simulink model "simVINS"  (R2018a)
settings: Solver=FixedStepDiscrete  StartTime=0.0  StopTime=inf  FixedStep=1/Fs  RelTol=1e-3  EnableMultiTasking=on
PreLoadFcn:
  | calibrateSFMA=false
  | modelDef = getModelDef(calibrateSFMA);
  | load VINS_bus_definitions.mat;
  | 
  | imuLocationMm = [6 -4.5 -16.8];
  | dejitter_on = true;
  | fidPosUncert = 0.01;
  | 
  | Fs = 1000;  % nominal IMU sampling rate (Hz)
  | 
  | gyroCalBiases = [0;0;0];
  | gyroCalMatrix = eye(3);
  | gyroGsensMatrix = zeros(3,3);
  | Hgyro = [1 0 0 0; 0 1 0 0; 0 0 1 0];
  | 
  | accelCalBiases = [0;0;0];
  | accelCalMatrix = eye(3);
  | Haccel = [1 0 0 0; 0 1 0 0; 0 0 1 0];
  | 
  | imuPar = getImuPar('lmvpCalibrated');
  | optical_cal = getOpticalCalfile();
  | 
  | lastUsedMgyr = zeros(3,3);
  | 
  | 
  | 
  | simData = true;
  | if simData
  |    load truthTrajectory.mat;
  | 
  |    % set Fs based on the timestamps
  |    Fs = 1/mean(diff(truthTrajectory.t.Data));
  |    if Fs>990
  |      Fs = Fs/2;  % bring 1000 Hz down to 500 Hz for faster simulation
  |    end
  | end
  | 
  | imageTensor = uint8(zeros(384,384,2));
  | imageTstamps = 0;
  | useImages = false;
  | useFeatures = false;
  | imageFeatureMatrix = zeros(10,263);
  | 
  | bundle_num_points = 400;
  | bundle_num_frames = 60;
  | 
  | % get rid of following lines if no longer using global data stores to send truth data into VINS
  | truthTraj = Simulink.Signal;
  | truthTraj.DataType = 'Bus: truthTrajectoryBus';
  | truthTraj.InitialValue = '0';
  | truthTraj.Complexity = 'Real';
StartFcn:
  | cd 'C:\Users\efoxlin\Documents\MATLAB\VINS';
undefined symbols (not defined in the file or in its folder): accels, gyros, jumpToXyz, jumpToYaw, tstamp_imu_us, tstamp_vidcap_us, xyz, yaw
libraries: simulink x6, dspmtrx3 x6, dspsrcs4 x6, vrlib x5, dspsigops x2, dspstat3 x2, realtime_pacer_lib x1, dspswit3 x1
(part 1 of 2)
settings Model: Creator=Eric  LastModifiedBy=efoxlin
settings SolverCC: PositivePriorityOrder=on
settings OptimizationCC: DefaultParameterBehavior=Inlined  UseFloatMulNetSlope=on  DefaultUnderspecifiedDataType=single  EnhancedBackFolding=on  PassReuseOutputArgsAs=Individual arguments  EfficientFloat2IntCast=on  MaxStackSize=64  OptimizeBlockOrder=speed  DifferentSizesBufferReuse=on  OptimizationCustomize=off
settings DebuggingCC: SignalInfNanChecking=error  ReadBeforeWriteMsg=DisableAll  WriteAfterWriteMsg=DisableAll  WriteAfterReadMsg=DisableAll  CheckMatrixSingularityMsg=error  ParameterTunabilityLossMsg=error  UnderSpecifiedDataTypeMsg=warning  SignalLabelMismatchMsg=error  UnconnectedOutputMsg=none  BusObjectLabelMismatch=error
settings HardwareCC: ProdBitPerPointer=32  ProdBitPerSizeT=32  ProdBitPerPtrDiffT=32  ProdLargestAtomicInteger=Long  ProdLargestAtomicFloat=Double  ProdWordSize=32  ProdHWDeviceType=ARM Compatible->ARM Cortex
settings SFSimCC: SimParseCustomCode=off  MATLABDynamicMemAlloc=off
settings RTWCC: SystemTargetFile=ert.tlc  GenCodeOnly=on  TemplateMakefile=ert_default_tmf  GenerateReport=on  Toolchain=Microsoft Visual C++ 2017 v15.0 | nmake (64-bit Windows)  BuildConfiguration=Faster Runs  IncludeHyperlinkInReport=on  LaunchReport=on  TargetLang=C++  GenerateTraceInfo=on  GenerateTraceReport=on  GenerateTraceReportSl=on  GenerateTraceReportSf=on  GenerateTraceReportEml=on
settings CodeAppCC: ForceParamTrailComments=on  IgnoreCustomStorageClasses=off  OperatorAnnotations=on  SimulinkDataObjDesc=on  SFDataObjDesc=on  InsertBlockDesc=on
settings ERTTargetCC: TargetLangStandard=C++03 (ISO)  GenerateSampleERTMain=on  MultiInstanceERTCode=on  CodeInterfacePackaging=C++ class  InlinedParameterPlacement=NonHierarchical  RootIOFormat=Structure reference  ERTCustomFileTemplate=example_file_process.tlc

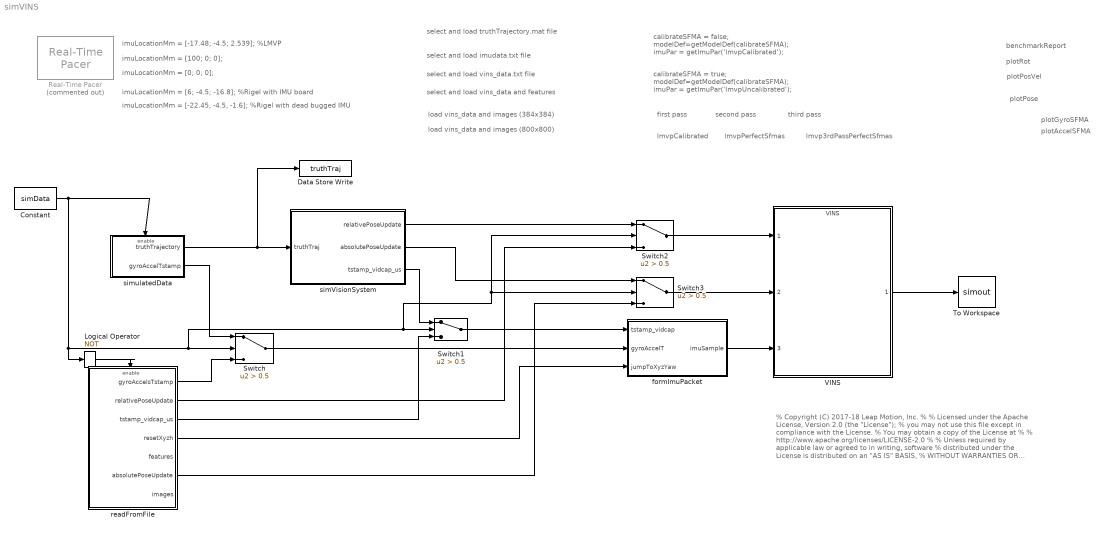
== system simVINS ==
  note: calibrateSFMA = false;
      | modelDef=getModelDef(calibrateSFMA);
      | imuPar = getImuPar('lmvpCalibrated');
  note: imuLocationMm = [-17.48; -4.5; 2.539]; %LMVP
  note: select and load imudata.txt file
  note: second pass
  note: first pass
  note: plotPosVel
  note: plotRot
  note: third pass
  note: select and load truthTrajectory.mat file
  note: lmvpCalibrated
  note: imuLocationMm = [0; 0; 0];
  note: imuLocationMm = [100; 0; 0];
  note: plotPose
  note: lmvpPerfectSfmas
  note: select and load vins_data.txt file
  note: lmvp3rdPassPerfectSfmas
  note: benchmarkReport
  note: calibrateSFMA = true;
      | modelDef=getModelDef(calibrateSFMA);
      | imuPar = getImuPar('lmvpUncalibrated');
  note: plotGyroSFMA
  note: plotAccelSFMA
  note: imuLocationMm = [6; -4.5; -16.8]; %Rigel with IMU board
  note: imuLocationMm = [-22.45, -4.5, -1.6]; %Rigel with dead bugged IMU
  note: select and load vins_data and features
  note: load vins_data and images (800x800)
  note: load vins_data and images (384x384)
  note: % Copyright (C) 2017-18 Leap Motion, Inc.
      | %
      | %    Licensed under the Apache License, Version 2.0 (the "License");
      | %    you may not use this file except in compliance with the License.
      | %    You may obtain a copy of the License at
      | %
      | %        http://www.apache.org/licenses/LICENSE-2.0
      | %
      | %    Unless required by applicable law or agreed to in writing, software
      | %    distributed under the License is distributed on an "AS IS" BASIS,
      | %    WITHOUT WARRANTIES OR CONDITIONS OF ANY KIND, either express or implied.
      | %    See the License for the specific language governing permissions and
      | %    limitations under the License.
      | % Author: Eric Foxlin
  Constant : Constant  Value=simData
  Data Store Write : DataStoreWrite  DataStoreName=truthTraj  DataStoreElements=truthTraj
  Logical Operator : Logic  Operator=NOT  IconShape=distinctive  AllPortsSameDT=off  OutDataTypeStr=boolean
  Real-Time Pacer : realtime_pacer_lib/Real-Time Pacer  Commented=on  simTimePerRealTime=1
  Switch{,1..3} (4 alike) : Switch  Criteria=u2 > Threshold  Threshold=0.5
  To Workspace : ToWorkspace  VariableName=simout  SaveFormat=Timeseries  SampleTime=-1
      settings: Save2DSignal=2-D array (concatenate along first dimension)
  VINS : ModelReference  ModelNameDialog=VINS.slx  SimulationMode=Normal  CodeInterface=Top model  ModelReferenceVersion=1.743
  formImuPacket : Subsystem
  readFromFile : Subsystem
  simVisionSystem : Subsystem  TreatAsAtomicUnit=on
  simulatedData : Subsystem
  wires:
  VINS/1 -> To Workspace/1
  readFromFile/1(gyroAccelsTstamp) -> Switch/3
  simulatedData/2("gyroAccelTstamp ") -> Switch/1
  Constant/1 -> Logical Operator/1, Switch2/2, Switch3/2, Switch1/2, Switch/2, simulatedData/Enable
  Logical Operator/1 -> readFromFile/Enable
  simulatedData/1(truthTrajectory) -> Data Store Write/1, simVisionSystem/1(truthTraj)
  Switch/1 -> formImuPacket/2(gyroAccelT)
  formImuPacket/1(imuSample) -> VINS/3
  simVisionSystem/3(tstamp_vidcap_us) -> Switch1/1
  simVisionSystem/1(relativePoseUpdate) -> Switch2/1
  Switch3/1 -> VINS/2
  Switch1/1 -> formImuPacket/1(tstamp_vidcap)
  readFromFile/3(tstamp_vidcap_us) -> Switch1/3
  Switch2/1 -> VINS/1
  readFromFile/2(relativePoseUpdate) -> Switch2/3
  readFromFile/4(resetXyzh) -> formImuPacket/3(jumpToXyzYaw)
  simVisionSystem/2(absolutePoseUpdate) -> Switch3/1
  readFromFile/6(absolutePoseUpdate) -> Switch3/3

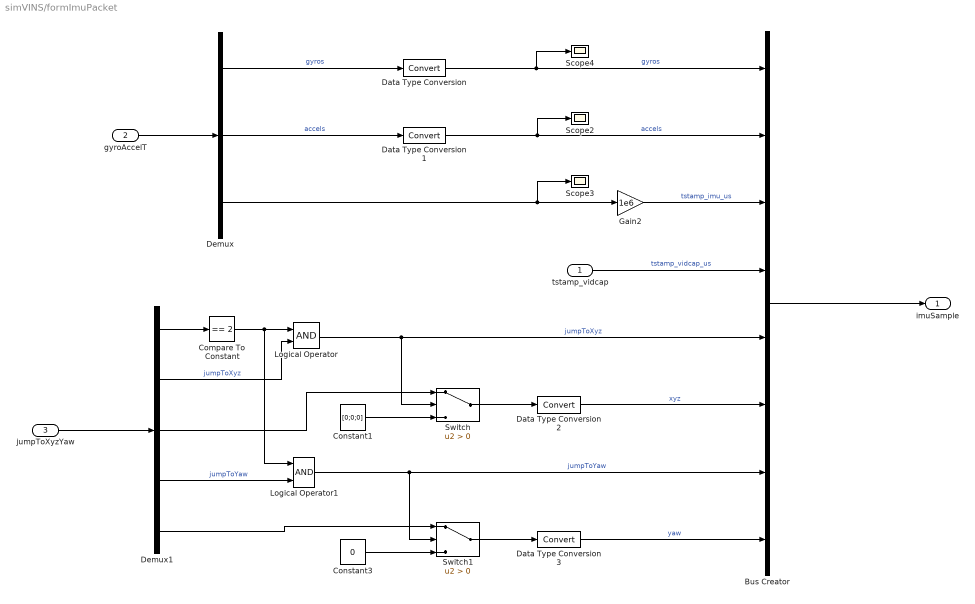
== system simVINS/formImuPacket ==
  tstamp_vidcap : Inport
  gyroAccelT : Inport  Port=2
  jumpToXyzYaw : Inport  Port=3
  Bus Creator : BusCreator  Inputs=gyros,accels,tstamp_imu_us,tstamp_vidcap_us,jumpToXyz,xyz,jumpToYaw,yaw  OutDataTypeStr=Bus: imuSample  NonVirtualBus=on
  Compare To Constant : simulink/Logic and Bit Operations/Compare To Constant  relop===  const=2  OutDataTypeStr=boolean
  Constant1 : Constant  Value=[0;0;0]
  Constant3 : Constant  Value=0
  Data Type Conversion{,1..3} (4 alike) : DataTypeConversion
  Demux : Demux  Outputs=[3 3 1]
  Demux1 : Demux  Outputs=[1 1 3 1 1]
  Gain2 : Gain  Gain=1e6
  Logical Operator : Logic  AllPortsSameDT=off  OutDataTypeStr=boolean
  Logical Operator1 : Logic  AllPortsSameDT=off  OutDataTypeStr=boolean
  Scope2 : Scope
  Scope3 : Scope
  Scope4 : Scope
  Switch : Switch  Criteria=u2 > Threshold
  Switch1 : Switch  Criteria=u2 > Threshold
  imuSample : Outport
  wires:
  Demux/2 -> Data Type Conversion1/1  "accels"
  Demux/1 -> Data Type Conversion/1  "gyros"
  gyroAccelT/1 -> Demux/1
  Bus Creator/1 -> imuSample/1
  Gain2/1 -> Bus Creator/3  "tstamp_imu_us"
  tstamp_vidcap/1 -> Bus Creator/4  "tstamp_vidcap_us"
  Data Type Conversion/1 -> Scope4/1, Bus Creator/1  "gyros"
  Data Type Conversion1/1 -> Scope2/1, Bus Creator/2  "accels"
  Demux/3 -> Gain2/1, Scope3/1
  Logical Operator/1 -> Switch/2, Bus Creator/5  "jumpToXyz"
  Data Type Conversion2/1 -> Bus Creator/6  "xyz"
  Logical Operator1/1 -> Switch1/2, Bus Creator/7  "jumpToYaw"
  Data Type Conversion3/1 -> Bus Creator/8  "yaw"
  jumpToXyzYaw/1 -> Demux1/1
  Demux1/1 -> Compare To Constant/1
  Demux1/2 -> Logical Operator/2  "jumpToXyz"
  Compare To Constant/1 -> Logical Operator1/1, Logical Operator/1
  Demux1/4 -> Logical Operator1/2  "jumpToYaw"
  Demux1/3 -> Switch/1
  Switch/1 -> Data Type Conversion2/1
  Constant1/1 -> Switch/3
  Switch1/1 -> Data Type Conversion3/1
  Demux1/5 -> Switch1/1
  Constant3/1 -> Switch1/3

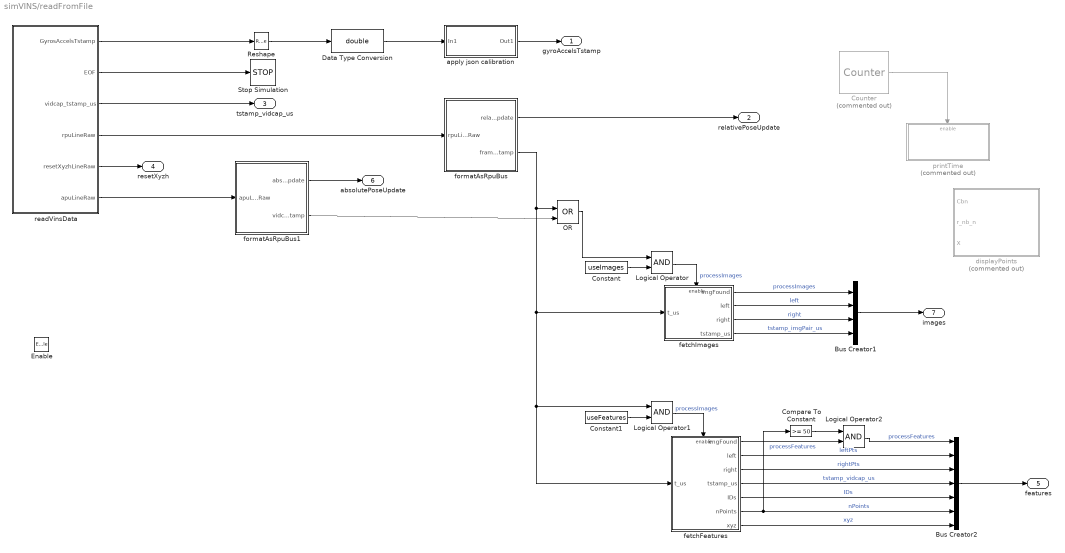
== system simVINS/readFromFile ==
  Enable : EnablePort
  Bus Creator1 : BusCreator  Inputs=4
  Bus Creator2 : BusCreator  Inputs=7
  Compare To Constant : simulink/Logic and Bit Operations/Compare To Constant  relop=>=  const=50  OutDataTypeStr=boolean
  Constant : Constant  Value=useImages
  Constant1 : Constant  Value=useFeatures
  Counter : dspswit3/Counter  Commented=on  Direction=Up  CountEvent=Free running  CounterSize=User defined  MaxCount=4095  InitialCount=0  Output=Hit  HitValue=32  ResetInput=off  SamplesPerFrame=1  Ts=1/Fs  CntDtype=double  HitDtype=Logical
  Data Type Conversion : DataTypeConversion  OutDataTypeStr=double
  Logical Operator : Logic  AllPortsSameDT=off  OutDataTypeStr=boolean
  Logical Operator1 : Logic  AllPortsSameDT=off  OutDataTypeStr=boolean
  Logical Operator2 : Logic  AllPortsSameDT=off  OutDataTypeStr=boolean
  OR : Logic  Operator=OR  IconShape=distinctive  AllPortsSameDT=off  OutDataTypeStr=boolean
  Reshape : Reshape  OutputDimensionality=Column vector (2-D)
  Stop Simulation : Stop
  apply json calibration : Subsystem  TreatAsAtomicUnit=on
  displayPoints : MATLAB Function  Commented=on  TreatAsAtomicUnit=on
  fetchFeatures : Subsystem
  fetchImages : Subsystem
  formatAsRpuBus : Subsystem
  formatAsRpuBus1 : Subsystem
  printTime : Subsystem  Commented=on
  readVinsData : Subsystem
  gyroAccelsTstamp : Outport
  relativePoseUpdate : Outport  Port=2
  tstamp_vidcap_us : Outport  Port=3
  resetXyzh : Outport  Port=4
  features : Outport  Port=5
  absolutePoseUpdate : Outport  Port=6
  images : Outport  Port=7
  wires:
  Reshape/1 -> Data Type Conversion/1
  readVinsData/1(GyrosAccelsTstamp) -> Reshape/1
  readVinsData/2(EOF) -> Stop Simulation/1
  Data Type Conversion/1 -> apply json calibration/1(In1)
  Counter/1 -> printTime/Enable
  apply json calibration/1(Out1) -> gyroAccelsTstamp/1
  readVinsData/3(vidcap_tstamp_us) -> tstamp_vidcap_us/1
  readVinsData/5(resetXyzhLineRaw) -> resetXyzh/1
  fetchImages/2(left) -> Bus Creator1/2  "left"
  fetchImages/3(right) -> Bus Creator1/3  "right"
  Constant/1 -> Logical Operator/2
  Bus Creator1/1 -> images/1
  fetchImages/1(imgFound) -> Bus Creator1/1  "processImages"
  fetchImages/4(tstamp_us) -> Bus Creator1/4  "tstamp_imgPair_us"
  OR/1 -> Logical Operator/1
  readVinsData/4(rpuLineRaw) -> formatAsRpuBus/1(rpuLineRaw)
  formatAsRpuBus/1(relativePoseUpdate) -> relativePoseUpdate/1
  readVinsData/6(apuLineRaw) -> formatAsRpuBus1/1(apuLineRaw)
  formatAsRpuBus1/2(vidcap tstamp) -> OR/2
  Logical Operator/1 -> fetchImages/Enable  "processImages"
  formatAsRpuBus1/1(absolutePoseUpdate) -> absolutePoseUpdate/1
  Logical Operator1/1 -> fetchFeatures/Enable  "processImages"
  formatAsRpuBus/2(frame2 tstamp) -> fetchImages/1(t_us), Logical Operator1/1, fetchFeatures/1(t_us), OR/1
  Constant1/1 -> Logical Operator1/2
  Logical Operator2/1 -> Bus Creator2/1  "processFeatures"
  fetchFeatures/2(left) -> Bus Creator2/2  "leftPts"
  fetchFeatures/3(right) -> Bus Creator2/3  "rightPts"
  fetchFeatures/4(tstamp_us) -> Bus Creator2/4  "tstamp_vidcap_us"
  Bus Creator2/1 -> features/1
  fetchFeatures/5(IDs) -> Bus Creator2/5  "IDs"
  fetchFeatures/6(nPoints) -> Compare To Constant/1, Bus Creator2/6  "nPoints"
  fetchFeatures/7(xyz) -> Bus Creator2/7  "xyz"
  fetchFeatures/1(imgFound) -> Logical Operator2/2  "processFeatures"
  Compare To Constant/1 -> Logical Operator2/1

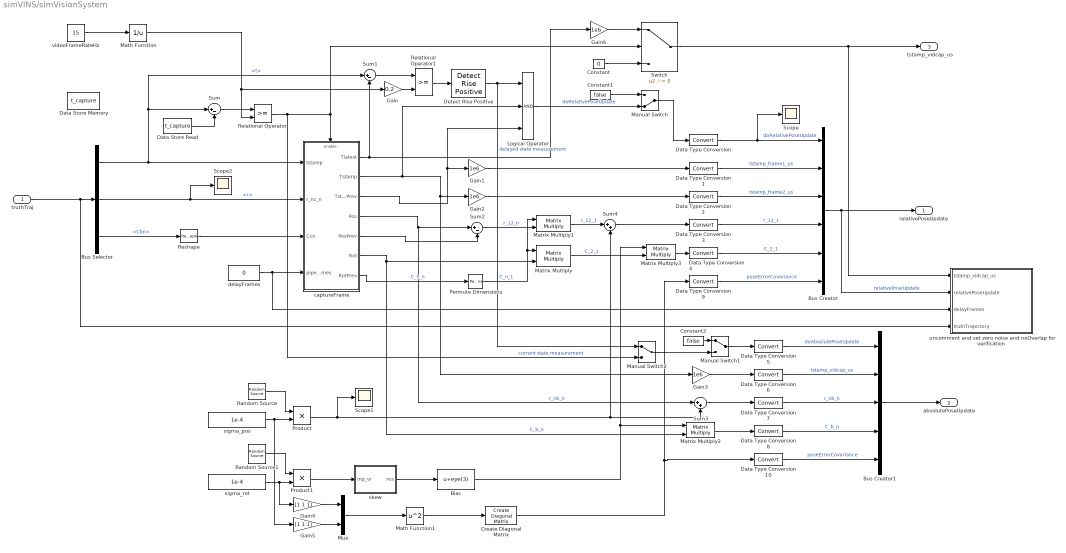
== system simVINS/simVisionSystem ==
  truthTraj : Inport
  Bias : Bias  Bias=eye(3)
  Bus Creator : BusCreator  Inputs=6  OutDataTypeStr=Bus: relativePoseUpdate  NonVirtualBus=on
  Bus Creator1 : BusCreator  Inputs=5  OutDataTypeStr=Bus: absolutePoseUpdate  NonVirtualBus=on
  Bus Selector : BusSelector  OutputSignals=t,r,Cbn
  Constant : Constant  Value=0
  Constant1 : Constant  Value=false
  Constant2 : Constant  Value=false
  Create Diagonal Matrix : dspmtrx3/Create Diagonal Matrix
      settings: SourceProductName=DSP System Toolbox  SourceProductBaseCode=DS
  Data Store Memory : DataStoreMemory  DataStoreName=t_capture  ReadBeforeWriteMsg=warning  WriteAfterWriteMsg=warning  WriteAfterReadMsg=warning  ShowAdditionalParam=off
  Data Store Read : DataStoreRead  DataStoreName=t_capture
  Data Type Conversion{,1..10} (11 alike) : DataTypeConversion
  Detect Rise Positive : simulink/Logic and Bit Operations/Detect Rise Positive  vinit=0  OutDataTypeStr=boolean
  Gain : Gain  Gain=0.2
  Gain{1..3,6} (4 alike) : Gain  Gain=1e6
  Gain4 : Gain  Gain=[1 1 1]
  Gain5 : Gain  Gain=[1 1 1]
  Logical Operator : Logic  Inputs=3  AllPortsSameDT=off  OutDataTypeStr=boolean
  Manual Switch : ManualSwitch  CurrentSetting=0
  Manual Switch1 : ManualSwitch
  Manual Switch2 : ManualSwitch
  Math Function : Math  Operator=reciprocal  SaturateOnIntegerOverflow=on
  Math Function1 : Math  Operator=square  SaturateOnIntegerOverflow=on
  Matrix Multiply{,1..3} (4 alike) : Product  Multiplication=Matrix(*)
  Mux : Mux  Inputs=2
  Permute Dimensions : PermuteDimensions
  Product : Product
  Product1 : Product
  Random Source : dspsrcs4/Random Source  SrcType=Gaussian  NormMethod=Ziggurat  CltLength=12  MinVal=0  MaxVal=1  MeanVal=[0; 0 ; 0]  VarVal=1  RepMode=Not repeatable  rawSeed=1  IsInherit=off  SampMode=Discrete  SampTime=1/Fs  SampFrame=1  DataType=Double  OutComplex=Real  OutputFrames=off
  Random Source1 : dspsrcs4/Random Source  SrcType=Gaussian  NormMethod=Ziggurat  CltLength=12  MinVal=0  MaxVal=1  MeanVal=[0; 0 ; 0]  VarVal=1  RepMode=Not repeatable  rawSeed=1  IsInherit=off  SampMode=Discrete  SampTime=1/Fs  SampFrame=1  DataType=Double  OutComplex=Real  OutputFrames=off
  Relational Operator : RelationalOperator  OutDataTypeStr=boolean  RndMeth=Simplest
  Relational Operator1 : RelationalOperator  OutDataTypeStr=boolean  RndMeth=Simplest
  Reshape : Reshape  OutputDimensionality=Customize  OutputDimensions=[3,3]
  Scope : Scope
  Scope1 : Scope
  Scope2 : Scope
  Sum : Sum  Inputs=|+-
  Sum1 : Sum  Inputs=|+-
  Sum2 : Sum  Inputs=|+-
  Sum3 : Sum  Inputs=|++
  Sum4 : Sum  Inputs=|++
  Switch : Switch  Criteria=u2 ~= 0
  captureFrame : Subsystem  TreatAsAtomicUnit=on
  delayFrames : Constant  Value=0
  sigma_pos : Constant  Value=1e-4
  sigma_rot : Constant  Value=1e-4
  skew : MATLAB Function  TreatAsAtomicUnit=on
  uncomment and set zero noise and noOverlap for verification : Subsystem  TreatAsAtomicUnit=on
  videoFrameRateHz : Constant  Value=15
  relativePoseUpdate : Outport
  absolutePoseUpdate : Outport  Port=2
  tstamp_vidcap_us : Outport  Port=3
  wires:
  truthTraj/1 -> uncomment and set zero noise and noOverlap for verification/4(truthTrajectory), Bus Selector/1
  Bus Selector/1 -> Sum/1, Sum1/1, captureFrame/1(tstamp)  "<t>"
  Sum/1 -> Relational Operator/1
  videoFrameRateHz/1 -> Math Function/1
  Math Function/1 -> Relational Operator/2, Gain/1
  Relational Operator/1 -> Manual Switch2/2, Switch/2, captureFrame/Enable  "current state measurement"
  Bus Selector/2 -> Scope2/1, captureFrame/2(r_nc_n)  "<r>"
  Bus Selector/3 -> Reshape/1  "<Cbn>"
  captureFrame/4(Pos) -> Sum3/1, Sum2/1  "r_nb_n"
  captureFrame/6(Rot) -> Matrix Multiply2/2, Matrix Multiply/2  "C_b_n"
  Sum1/1 -> Relational Operator1/1
  Gain/1 -> Relational Operator1/2
  Relational Operator1/1 -> Detect Rise Positive/1
  captureFrame/3(TstampPrev) -> Logical Operator/3, Gain1/1
  Manual Switch/1 -> Data Type Conversion/1
  captureFrame/2(Tstamp) -> Logical Operator/2, Gain3/1, Gain2/1
  captureFrame/5(PosPrev) -> Sum2/2
  Sum2/1 -> Matrix Multiply1/2  "r_12_n"
  Reshape/1 -> captureFrame/3(Ccn)
  Matrix Multiply3/1 -> Data Type Conversion4/1
  captureFrame/7(RotPrev) -> Permute Dimensions/1  "C_1_n"
  Permute Dimensions/1 -> Matrix Multiply1/1, Matrix Multiply/1  "C_n_1"
  Bus Creator/1 -> relativePoseUpdate/1, uncomment and set zero noise and noOverlap for verification/2(relativePoseUpdate)  "relativePoseUpdate"
  Sum4/1 -> Data Type Conversion3/1
  Gain1/1 -> Data Type Conversion1/1
  Gain2/1 -> Data Type Conversion2/1
  Data Store Read/1 -> Sum/2
  Switch/1 -> tstamp_vidcap_us/1, uncomment and set zero noise and noOverlap for verification/1(tstamp_vidcap_us)
  Constant/1 -> Switch/3
  Detect Rise Positive/1 -> Logical Operator/1, Manual Switch2/1  "delayed state measurement"
  Logical Operator/1 -> Manual Switch/2  "doRelativePoseUpdate"
  Constant1/1 -> Manual Switch/1
  Bus Creator1/1 -> absolutePoseUpdate/1
  Constant2/1 -> Manual Switch1/1
  Manual Switch1/1 -> Data Type Conversion5/1
  Gain3/1 -> Data Type Conversion6/1
  Sum3/1 -> Data Type Conversion7/1
  Matrix Multiply2/1 -> Data Type Conversion8/1
  sigma_pos/1 -> Gain5/1, Product/2
  Random Source/1 -> Product/1
  Random Source1/1 -> Product1/1
  sigma_rot/1 -> Gain4/1, Product1/2
  Product1/1 -> skew/1(inp_vr)
  skew/1(res) -> Bias/1
  Manual Switch2/1 -> Manual Switch1/2
  Bias/1 -> Matrix Multiply3/1, Matrix Multiply2/1
  Matrix Multiply1/1 -> Sum4/1  "r_12_1"
  Matrix Multiply/1 -> Matrix Multiply3/2  "C_2_1"
  Data Type Conversion/1 -> Scope/1, Bus Creator/1  "doRelativePoseUpdate"
  Data Type Conversion1/1 -> Bus Creator/2  "tstamp_frame1_us"
  Data Type Conversion2/1 -> Bus Creator/3  "tstamp_frame2_us"
  Data Type Conversion3/1 -> Bus Creator/4  "r_12_1"
  Data Type Conversion4/1 -> Bus Creator/5  "C_2_1"
  Data Type Conversion5/1 -> Bus Creator1/1  "doAbsolutePoseUpdate"
  Data Type Conversion6/1 -> Bus Creator1/2  "tstamp_vidcap_us"
  Data Type Conversion7/1 -> Bus Creator1/3  "r_nb_n"
  Data Type Conversion8/1 -> Bus Creator1/4  "C_b_n"
  Gain4/1 -> Mux/1
  Gain5/1 -> Mux/2
  Mux/1 -> Math Function1/1
  Data Type Conversion9/1 -> Bus Creator/6  "poseErrorCovariance"
  Data Type Conversion10/1 -> Bus Creator1/5  "poseErrorCovariance"
  Create Diagonal Matrix/1 -> Data Type Conversion10/1, Data Type Conversion9/1
  Math Function1/1 -> Create Diagonal Matrix/1
  delayFrames/1 -> uncomment and set zero noise and noOverlap for verification/3(delayFrames), captureFrame/4(pipelineDelayFrames)
  captureFrame/1(Tlatest) -> Gain6/1, Sum1/2
  Gain6/1 -> Switch/1
  Product/1 -> Scope1/1, Sum4/2, Sum3/2

== system simVINS/simulatedData ==
  note: truthTrajectory is motion of the camera device frame with origin
      | halfway between two lenses.
      | VINS tracking is done in body frame of IMU, which is offset
      | by imuLocationMm,  but output is converted to device frame.
  Enable : EnablePort
  From Workspace : FromWorkspace  VariableName=truthTrajectory  OutDataTypeStr=Bus: truthTrajectoryBus  SampleTime=1/Fs  Interpolate=off  OutputAfterFinalValue=Setting to zero
  To Workspace1 : ToWorkspace  VariableName=truthout  SaveFormat=Timeseries  SampleTime=-1
      settings: Save2DSignal=2-D array (concatenate along first dimension)
  reportOutputs : Subsystem  Priority=10  TreatAsAtomicUnit=on
  simulateIdealImuWithOffset : Subsystem
  simulateImuErrors : Subsystem  TreatAsAtomicUnit=on
  "t, rpy, PQR, rnav, vnav, anav way too slow!" : FromFile  Commented=on  FileName=truthTrajectory.mat  OutDataTypeStr=Bus: truthTrajectoryBus  SampleTime=1/Fs  ExtrapolationBeforeFirstDataPoint=Ground value  InterpolationWithinTimeRange=Zero order hold  ExtrapolationAfterLastDataPoint=Ground value
  uncomment for INS integration verification : Subsystem  TreatAsAtomicUnit=on
  truthTrajectory : Outport
  "gyroAccelTstamp " : Outport  Port=2
  wires:
  simulateIdealImuWithOffset/1(gyrosAccelsTstamp) -> uncomment for INS integration verification/1(gyroAccelT), simulateImuErrors/1(gyroAccelT)
  From Workspace/1 -> truthTrajectory/1, reportOutputs/1(truthTraj), uncomment for INS integration verification/2(truthTrajectory), simulateIdealImuWithOffset/1(In1)
  reportOutputs/1(truthOut) -> To Workspace1/1
  simulateImuErrors/5(withErrors) -> "gyroAccelTstamp "/1
  simulateImuErrors/1(gyroBias) -> reportOutputs/2(truth dw)
  simulateImuErrors/2(accelBias) -> reportOutputs/3(truth df)

== system simVINS/readFromFile/apply json calibration ==
  note: if there is a .json file in the directory where imudata.txt file had been stored,
      | it gets parsed during file load to produce the homogeneous 3x4 matrices Hgyro and Haccel.
      | If not, these are set to identity with no biases so that they don't do anything.
  In1 : Inport
  Constant : Constant  Value=Hgyro
  Constant1 : Constant  Value=Haccel
  Demux : Demux  Outputs=[3 3 1]
  Mux : Mux  Inputs=3
  Product : Product  Multiplication=Matrix(*)
  Product1 : Product  Multiplication=Matrix(*)
  Reshape : Reshape  OutputDimensionality=Column vector (2-D)
  Reshape1 : Reshape  OutputDimensionality=Column vector (2-D)
  add a 1 as fourth element for homogeneous multiply : dspsigops/Pad  padAlong=Columns  dimsToPad=1  valSrc=Specify via dialog  padVal=1  spec=Output size  padNumOutRowsSpecMethod=User-specified  numOutRows=4  padNumOutColsSpecMethod=User-specified  numOutCols=1  isVarDimsMode=off  padBeginning=0  padEnd=0  outSizeMode=User-specified  outSize=1  padSigAt=End  trunc_flag=None  roundingMode=Floor  overflowMode=off  truncOrWrapMode=Truncate  wrap_flag=None
      settings: SourceProductName=DSP System Toolbox  SourceProductBaseCode=DS
  add a 1 as fourth element for homogeneous multiply1 : dspsigops/Pad  padAlong=Columns  dimsToPad=1  valSrc=Specify via dialog  padVal=1  spec=Output size  padNumOutRowsSpecMethod=User-specified  numOutRows=4  padNumOutColsSpecMethod=User-specified  numOutCols=1  isVarDimsMode=off  padBeginning=0  padEnd=0  outSizeMode=User-specified  outSize=1  padSigAt=End  trunc_flag=None  roundingMode=Floor  overflowMode=off  truncOrWrapMode=Truncate  wrap_flag=None
      settings: SourceProductName=DSP System Toolbox  SourceProductBaseCode=DS
  Out1 : Outport
  wires:
  In1/1 -> Demux/1
  Demux/1 -> Reshape/1
  Constant/1 -> Product/1
  Demux/2 -> Reshape1/1
  Constant1/1 -> Product1/1
  Product/1 -> Mux/1
  Product1/1 -> Mux/2
  Mux/1 -> Out1/1
  Reshape/1 -> add a 1 as fourth element for homogeneous multiply/1
  Reshape1/1 -> add a 1 as fourth element for homogeneous multiply1/1
  add a 1 as fourth element for homogeneous multiply/1 -> Product/2
  add a 1 as fourth element for homogeneous multiply1/1 -> Product1/2
  Demux/3 -> Mux/3

== system simVINS/readFromFile/fetchFeatures ==
  t_us : Inport
  Enable : EnablePort  PropagateVarSize=During execution
  Constant : Constant  Value=imageFeatureMatrix
  Display1 : Display
  MATLAB Function : MATLAB Function  TreatAsAtomicUnit=on
  Scope : Scope
  getImgNum : Subsystem  Priority=1
  imgFound : Outport  OutputWhenDisabled=reset  InitialOutput=false
  left : Outport  Port=2
  right : Outport  Port=3
  tstamp_us : Outport  Port=4  OutputWhenDisabled=reset  InitialOutput=0
  IDs : Outport  Port=5
  nPoints : Outport  Port=6
  xyz : Outport  Port=7
  wires:
  getImgNum/2(imgFound) -> imgFound/1
  t_us/1 -> getImgNum/1(t_us), tstamp_us/1
  MATLAB Function/4(rightPts) -> right/1
  Constant/1 -> MATLAB Function/2(imageFeatureMatrix)
  getImgNum/1(imgNum) -> Scope/1, MATLAB Function/1(imgNum)
  MATLAB Function/3(leftPts) -> left/1
  MATLAB Function/2(IDs) -> IDs/1
  MATLAB Function/1(nPoints) -> Display1/1, nPoints/1
  MATLAB Function/5(xyz) -> xyz/1

== system simVINS/readFromFile/fetchImages ==
  t_us : Inport
  Enable : EnablePort
  Constant : Constant  Value=imageTensor
  MATLAB Function : MATLAB Function  TreatAsAtomicUnit=on
  Scope : Scope
  getImgNum : Subsystem  Priority=1
  imgFound : Outport  OutputWhenDisabled=reset  InitialOutput=false
  left : Outport  Port=2
  right : Outport  Port=3
  tstamp_us : Outport  Port=4  OutputWhenDisabled=reset  InitialOutput=0
  wires:
  MATLAB Function/1(left) -> left/1
  getImgNum/1(imgNum) -> MATLAB Function/1(imgNum), Scope/1
  Constant/1 -> MATLAB Function/2(imageTensor)
  MATLAB Function/2(right) -> right/1
  t_us/1 -> tstamp_us/1, getImgNum/1(t_us)
  getImgNum/2(imgFound) -> imgFound/1

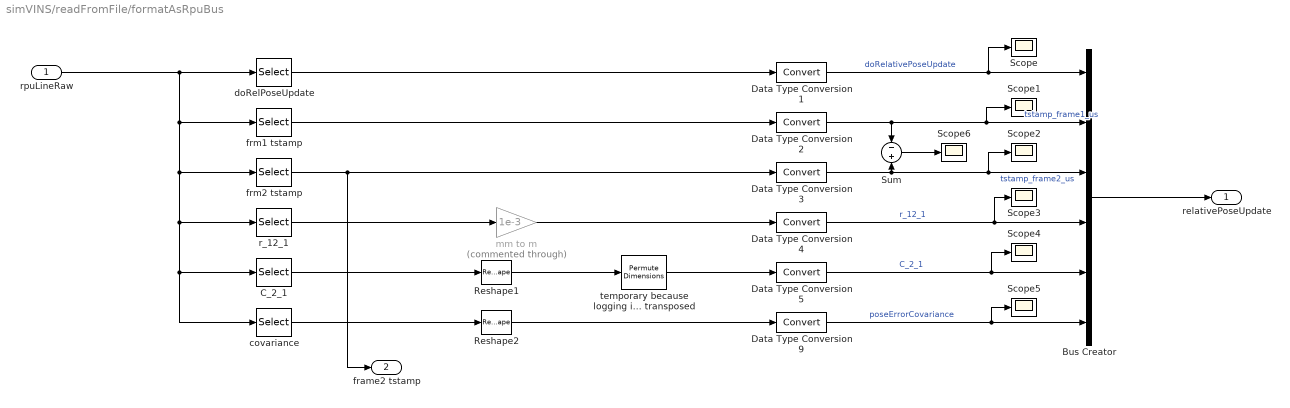
== system simVINS/readFromFile/formatAsRpuBus ==
  rpuLineRaw : Inport
  Bus Creator : BusCreator  Inputs=6  OutDataTypeStr=Bus: relativePoseUpdate  NonVirtualBus=on
  C_2_1 : Selector  InputPortWidth=52  IndexOptions=Index vector (dialog)  Indices=4:12  OutputSizes=1
  Data Type Conversion{1..5,9} (6 alike) : DataTypeConversion
  Reshape1 : Reshape  OutputDimensionality=Customize  OutputDimensions=[3,3]
  Reshape2 : Reshape  OutputDimensionality=Customize  OutputDimensions=[6,6]
  Scope{,1..6} (7 alike) : Scope
  Sum : Sum  Inputs=-+
  covariance : Selector  InputPortWidth=52  IndexOptions=Index vector (dialog)  Indices=16:51  OutputSizes=1
  doRelPoseUpdate : Selector  InputPortWidth=52  IndexOptions=Index vector (dialog)  Indices=52  OutputSizes=1
  frm1 tstamp : Selector  InputPortWidth=52  IndexOptions=Index vector (dialog)  Indices=2  OutputSizes=1
  frm2 tstamp : Selector  InputPortWidth=52  IndexOptions=Index vector (dialog)  Indices=3  OutputSizes=1
  mm to m : Gain  Commented=through  Gain=1e-3
  r_12_1 : Selector  InputPortWidth=52  IndexOptions=Index vector (dialog)  Indices=13:15  OutputSizes=1
  temporary because logging is transposed : PermuteDimensions
  relativePoseUpdate : Outport
  frame2 tstamp : Outport  Port=2
  wires:
  Sum/1 -> Scope6/1
  Data Type Conversion3/1 -> Sum/2, Bus Creator/3, Scope2/1  "tstamp_frame2_us"
  rpuLineRaw/1 -> frm1 tstamp/1, frm2 tstamp/1, r_12_1/1, C_2_1/1, covariance/1, doRelPoseUpdate/1
  Reshape1/1 -> temporary because logging is transposed/1
  C_2_1/1 -> Reshape1/1
  Data Type Conversion9/1 -> Scope5/1, Bus Creator/6  "poseErrorCovariance"
  doRelPoseUpdate/1 -> Data Type Conversion1/1
  Data Type Conversion2/1 -> Sum/1, Scope1/1, Bus Creator/2  "tstamp_frame1_us"
  Data Type Conversion5/1 -> Scope4/1, Bus Creator/5  "C_2_1"
  r_12_1/1 -> mm to m/1
  frm2 tstamp/1 -> frame2 tstamp/1, Data Type Conversion3/1
  Data Type Conversion1/1 -> Scope/1, Bus Creator/1  "doRelativePoseUpdate"
  temporary because logging is transposed/1 -> Data Type Conversion5/1
  Reshape2/1 -> Data Type Conversion9/1
  Data Type Conversion4/1 -> Scope3/1, Bus Creator/4  "r_12_1"
  frm1 tstamp/1 -> Data Type Conversion2/1
  covariance/1 -> Reshape2/1
  mm to m/1 -> Data Type Conversion4/1
  Bus Creator/1 -> relativePoseUpdate/1

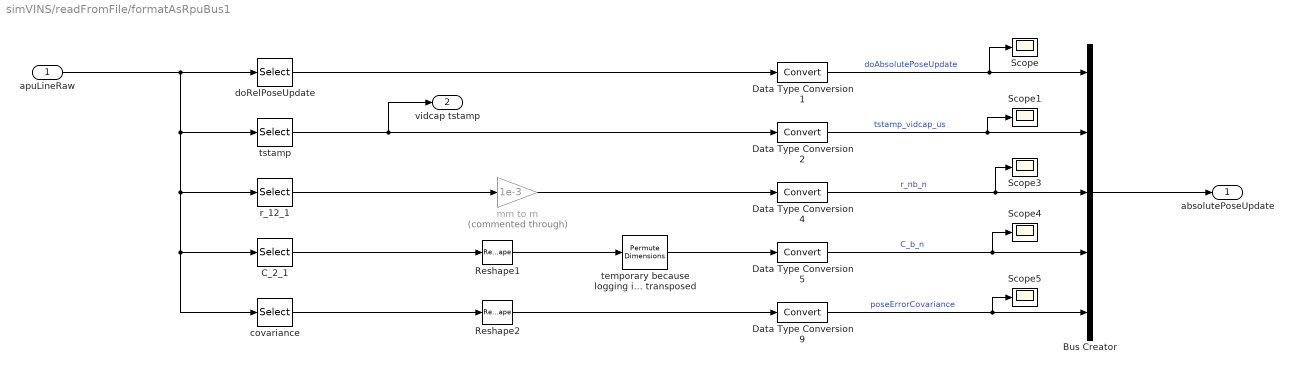
== system simVINS/readFromFile/formatAsRpuBus1 ==
  apuLineRaw : Inport
  " tstamp" : Selector  InputPortWidth=51  IndexOptions=Index vector (dialog)  Indices=2  OutputSizes=1
  Bus Creator : BusCreator  Inputs=5  OutDataTypeStr=Bus: absolutePoseUpdate  NonVirtualBus=on
  C_2_1 : Selector  InputPortWidth=51  IndexOptions=Index vector (dialog)  Indices=3:11  OutputSizes=1
  Data Type Conversion{1..2,4..5,9} (5 alike) : DataTypeConversion
  Reshape1 : Reshape  OutputDimensionality=Customize  OutputDimensions=[3,3]
  Reshape2 : Reshape  OutputDimensionality=Customize  OutputDimensions=[6,6]
  Scope{,1,3..5} (5 alike) : Scope
  covariance : Selector  InputPortWidth=51  IndexOptions=Index vector (dialog)  Indices=15:50  OutputSizes=1
  doRelPoseUpdate : Selector  InputPortWidth=51  IndexOptions=Index vector (dialog)  Indices=51  OutputSizes=1
  mm to m : Gain  Commented=through  Gain=1e-3
  r_12_1 : Selector  InputPortWidth=51  IndexOptions=Index vector (dialog)  Indices=12:14  OutputSizes=1
  temporary because logging is transposed : PermuteDimensions
  absolutePoseUpdate : Outport
  vidcap tstamp : Outport  Port=2
  wires:
  Bus Creator/1 -> absolutePoseUpdate/1
  mm to m/1 -> Data Type Conversion4/1
  covariance/1 -> Reshape2/1
  " tstamp"/1 -> vidcap tstamp/1, Data Type Conversion2/1
  Data Type Conversion4/1 -> Bus Creator/3, Scope3/1  "r_nb_n"
  Reshape2/1 -> Data Type Conversion9/1
  temporary because logging is transposed/1 -> Data Type Conversion5/1
  Data Type Conversion1/1 -> Bus Creator/1, Scope/1  "doAbsolutePoseUpdate"
  r_12_1/1 -> mm to m/1
  Data Type Conversion5/1 -> Bus Creator/4, Scope4/1  "C_b_n"
  Data Type Conversion2/1 -> Bus Creator/2, Scope1/1  "tstamp_vidcap_us"
  doRelPoseUpdate/1 -> Data Type Conversion1/1
  Data Type Conversion9/1 -> Bus Creator/5, Scope5/1  "poseErrorCovariance"
  C_2_1/1 -> Reshape1/1
  Reshape1/1 -> temporary because logging is transposed/1
  apuLineRaw/1 -> covariance/1, C_2_1/1, r_12_1/1, " tstamp"/1, doRelPoseUpdate/1

== system simVINS/readFromFile/printTime ==
  Enable : EnablePort
  Digital Clock : DigitalClock  SampleTime=1/Fs
  MATLAB Function : MATLAB Function  TreatAsAtomicUnit=on
  wires:
  Digital Clock/1 -> MATLAB Function/1(u)

== system simVINS/readFromFile/readVinsData ==
  C++ S-function : S-Function  FunctionName=readVinsData  Parameters=1/Fs  SFunctionDeploymentMode=off  EnableBusSupport=off
  Gain : Gain  Gain=1e-6
  Mux : Mux  Inputs=[3 3 1]
  Unit Delay : UnitDelay  SampleTime=-1
  accels : Selector  InputPortWidth=10  IndexOptions=Index vector (dialog)  Indices=3:5  OutputSizes=1
  avoid sending garbage on the last row : Switch  Criteria=u2 > Threshold  Threshold=0.5
  gyros : Selector  InputPortWidth=10  IndexOptions=Index vector (dialog)  Indices=6:8  OutputSizes=1
  t_us : Selector  InputPortWidth=10  IndexOptions=Index vector (dialog)  Indices=2  OutputSizes=1
  vidcap_tstamp : Selector  InputPortWidth=10  IndexOptions=Index vector (dialog)  Indices=9  OutputSizes=1
  GyrosAccelsTstamp : Outport
  EOF : Outport  Port=2
  vidcap_tstamp_us : Outport  Port=3
  rpuLineRaw : Outport  Port=4
  resetXyzhLineRaw : Outport  Port=5
  apuLineRaw : Outport  Port=6
  wires:
  C++ S-function/1 -> t_us/1, gyros/1, accels/1, vidcap_tstamp/1
  Mux/1 -> Unit Delay/1, avoid sending garbage on the last row/3
  avoid sending garbage on the last row/1 -> GyrosAccelsTstamp/1
  Unit Delay/1 -> avoid sending garbage on the last row/1
  C++ S-function/5 -> avoid sending garbage on the last row/2, EOF/1
  C++ S-function/2 -> rpuLineRaw/1
  vidcap_tstamp/1 -> vidcap_tstamp_us/1
  gyros/1 -> Mux/1
  accels/1 -> Mux/2
  t_us/1 -> Gain/1
  Gain/1 -> Mux/3
  C++ S-function/3 -> resetXyzhLineRaw/1
  C++ S-function/4 -> apuLineRaw/1

== system simVINS/simVisionSystem/captureFrame ==
  tstamp : Inport
  r_nc_n : Inport  Port=2
  Ccn : Inport  Port=3
  pipelineDelayFrames : Inport  Port=4
  Enable : EnablePort
  Data Store Write : DataStoreWrite  DataStoreName=t_capture
  Delay : Delay  DelayLengthSource=Input port
      settings: InputPortMap=u0,p1
  Delay1 : Delay  DelayLengthSource=Input port
      settings: InputPortMap=u0,p1
  Delay2 : Delay  DelayLengthSource=Input port
      settings: InputPortMap=u0,p1
  Unit Delay3 : UnitDelay  SampleTime=-1
  Unit Delay4 : UnitDelay  SampleTime=-1
  Unit Delay5 : UnitDelay  SampleTime=-1
  Tlatest : Outport
  Tstamp : Outport  Port=2
  TstampPrev : Outport  Port=3
  Pos : Outport  Port=4
  PosPrev : Outport  Port=5
  Rot : Outport  Port=6
  RotPrev : Outport  Port=7
  wires:
  tstamp/1 -> Data Store Write/1, Delay/1, Tlatest/1
  Ccn/1 -> Delay2/1  "Cbn"
  Delay/1 -> Unit Delay3/1, Tstamp/1
  Unit Delay3/1 -> TstampPrev/1
  r_nc_n/1 -> Delay1/1
  Delay1/1 -> Unit Delay4/1, Pos/1
  Unit Delay4/1 -> PosPrev/1
  Delay2/1 -> Unit Delay5/1, Rot/1
  Unit Delay5/1 -> RotPrev/1
  pipelineDelayFrames/1 -> Delay2/2, Delay1/2, Delay/2

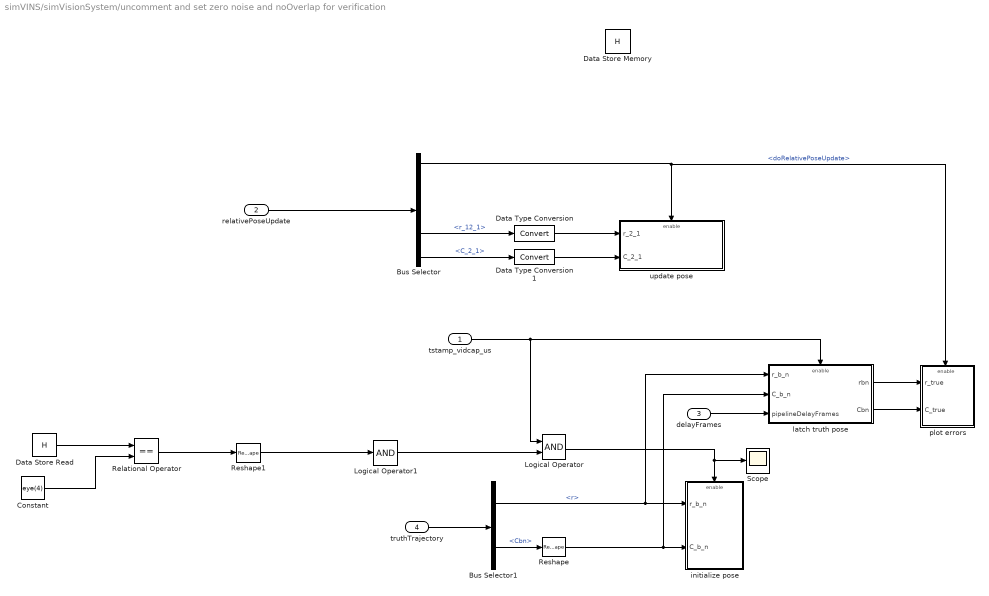
== system simVINS/simVisionSystem/uncomment and set zero noise and noOverlap for verification ==
  tstamp_vidcap_us : Inport
  relativePoseUpdate : Inport  Port=2
  delayFrames : Inport  Port=3
  truthTrajectory : Inport  Port=4
  Bus Selector : BusSelector  OutputSignals=doRelativePoseUpdate,tstamp_frame1_us,tstamp_frame2_us,r_12_1,C_2_1
  Bus Selector1 : BusSelector  OutputSignals=r,Cbn
  Constant : Constant  Value=eye(4)
  Data Store Memory : DataStoreMemory  DataStoreName=H  ReadBeforeWriteMsg=warning  WriteAfterWriteMsg=warning  WriteAfterReadMsg=warning  InitialValue=eye(4)  ShowAdditionalParam=off
  Data Store Read : DataStoreRead  DataStoreName=H
  Data Type Conversion : DataTypeConversion
  Data Type Conversion1 : DataTypeConversion
  Logical Operator : Logic  AllPortsSameDT=off  OutDataTypeStr=boolean
  Logical Operator1 : Logic  Inputs=1  AllPortsSameDT=off  OutDataTypeStr=boolean
  Relational Operator : RelationalOperator  Operator===  OutDataTypeStr=boolean  RndMeth=Simplest
  Reshape : Reshape  OutputDimensionality=Customize  OutputDimensions=[3,3]
  Reshape1 : Reshape
  Scope : Scope
  initialize pose : Subsystem  TreatAsAtomicUnit=on
  latch truth pose : Subsystem  TreatAsAtomicUnit=on
  plot errors : Subsystem  TreatAsAtomicUnit=on
  update pose : Subsystem  TreatAsAtomicUnit=on
  wires:
  relativePoseUpdate/1 -> Bus Selector/1
  Bus Selector/1 -> plot errors/Enable, update pose/Enable  "<doRelativePoseUpdate>"
  Bus Selector/4 -> Data Type Conversion/1  "<r_12_1>"
  Bus Selector/5 -> Data Type Conversion1/1  "<C_2_1>"
  truthTrajectory/1 -> Bus Selector1/1
  Bus Selector1/1 -> latch truth pose/1(r_b_n), initialize pose/1(r_b_n)  "<r>"
  Bus Selector1/2 -> Reshape/1  "<Cbn>"
  Logical Operator/1 -> Scope/1, initialize pose/Enable
  Data Store Read/1 -> Relational Operator/1
  Constant/1 -> Relational Operator/2
  Relational Operator/1 -> Reshape1/1
  tstamp_vidcap_us/1 -> latch truth pose/Enable, Logical Operator/1
  Reshape/1 -> latch truth pose/2(C_b_n), initialize pose/2(C_b_n)
  latch truth pose/1(rbn) -> plot errors/1(r_true)
  latch truth pose/2(Cbn) -> plot errors/2(C_true)
  Data Type Conversion/1 -> update pose/1(r_2_1)
  Data Type Conversion1/1 -> update pose/2(C_2_1)
  Logical Operator1/1 -> Logical Operator/2
  Reshape1/1 -> Logical Operator1/1
  delayFrames/1 -> latch truth pose/3(pipelineDelayFrames)

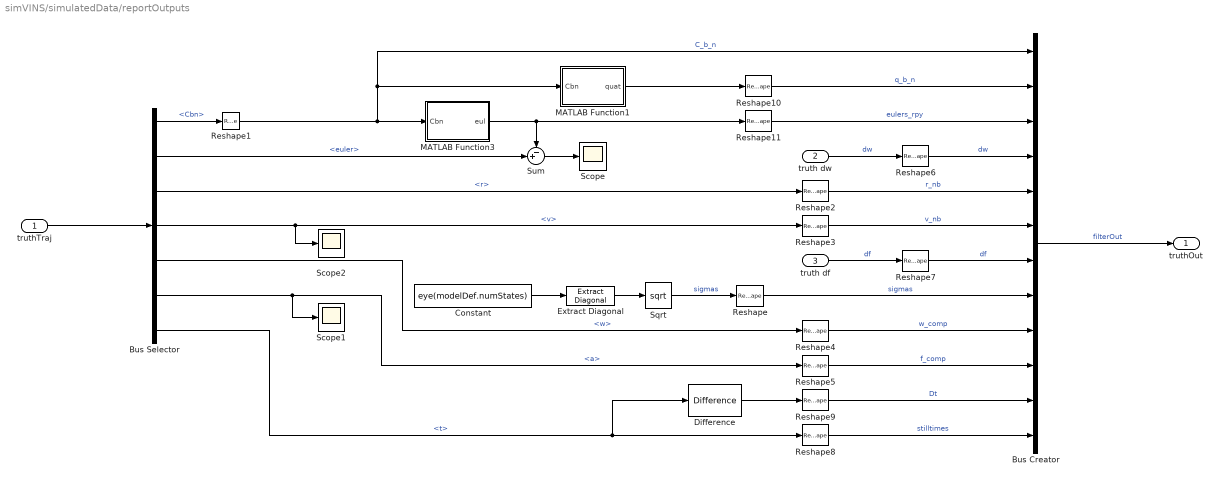
== system simVINS/simulatedData/reportOutputs ==
  truthTraj : Inport
  truth dw : Inport  Port=2
  truth df : Inport  Port=3
  Bus Creator : BusCreator  Inputs=12
  Bus Selector : BusSelector  OutputSignals=Cbn,euler,r,v,w,a,t
  Constant : Constant  Value=eye(modelDef.numStates)
  Difference : simulink/Discrete/Difference  ICPrevInput=0.0  OutMin=[]  OutMax=[]  OutDataType=fixdt(1, 16)  OutScaling=2^-10  DoSatur=off
  Extract Diagonal : dspmtrx3/Extract Diagonal
      settings: SourceProductName=DSP System Toolbox  SourceProductBaseCode=DS
  MATLAB Function1 : MATLAB Function  TreatAsAtomicUnit=on
  MATLAB Function3 : MATLAB Function  TreatAsAtomicUnit=on
  Reshape{,2..11} (11 alike) : Reshape  OutputDimensionality=Column vector (2-D)
  Reshape1 : Reshape  OutputDimensionality=Customize  OutputDimensions=[3,3]
  Scope : Scope
  Scope1 : Scope
  Scope2 : Scope
  Sqrt : Sqrt  SaturateOnIntegerOverflow=on
  Sum : Sum  Inputs=-+|
  truthOut : Outport
  wires:
  Reshape/1 -> Bus Creator/8  "sigmas"
  Bus Selector/7 -> Difference/1, Reshape8/1  "<t>"
  Reshape9/1 -> Bus Creator/11  "Dt"
  MATLAB Function1/1(quat) -> Reshape10/1
  MATLAB Function3/1(eul) -> Sum/1, Reshape11/1
  Bus Selector/3 -> Reshape2/1  "<r>"
  truth dw/1 -> Reshape6/1  "dw"
  Reshape3/1 -> Bus Creator/6  "v_nb"
  Reshape4/1 -> Bus Creator/9  "w_comp"
  truth df/1 -> Reshape7/1  "df"
  Reshape5/1 -> Bus Creator/10  "f_comp"
  Sqrt/1 -> Reshape/1  "sigmas"
  Bus Creator/1 -> truthOut/1  "filterOut"
  Constant/1 -> Extract Diagonal/1
  Extract Diagonal/1 -> Sqrt/1
  Reshape1/1 -> MATLAB Function3/1(Cbn), MATLAB Function1/1(Cbn), Bus Creator/1  "C_b_n"
  truthTraj/1 -> Bus Selector/1
  Bus Selector/1 -> Reshape1/1  "<Cbn>"
  Bus Selector/2 -> Sum/2  "<euler>"
  Reshape2/1 -> Bus Creator/5  "r_nb"
  Bus Selector/4 -> Scope2/1, Reshape3/1  "<v>"
  Sum/1 -> Scope/1
  Bus Selector/5 -> Reshape4/1  "<w>"
  Bus Selector/6 -> Scope1/1, Reshape5/1  "<a>"
  Reshape6/1 -> Bus Creator/4  "dw"
  Reshape7/1 -> Bus Creator/7  "df"
  Reshape8/1 -> Bus Creator/12  "stilltimes"
  Difference/1 -> Reshape9/1
  Reshape10/1 -> Bus Creator/2  "q_b_n"
  Reshape11/1 -> Bus Creator/3  "eulers_rpy"

== system simVINS/simulatedData/simulateIdealImuWithOffset ==
  In1 : Inport
  Bus Selector1 : BusSelector  OutputSignals=w,Cbn,a,wDot,t
  Constant : Constant  Value=imuLocationMm/1000
  Logical Operator : Logic  Operator=NOR  Inputs=1  AllPortsSameDT=off  OutDataTypeStr=boolean
  Mux1 : Mux  Inputs=3
  Permute Dimensions1 : PermuteDimensions
  Product : Product  Multiplication=Matrix(*)
  Reshape : Reshape  OutputDimensionality=Customize  OutputDimensions=[3,3]
  Scope{1..4} (4 alike) : Scope
  Stop Simulation : Stop
  Unit Delay : UnitDelay  SampleTime=-1
  avoid sending garbage on the last row : Switch  Criteria=u2 > Threshold  Threshold=0.5
  centripetalTangential : Subsystem  TreatAsAtomicUnit=on
  f = a-g : Bias  Bias=-[0;0;9.80665]
  gyrosAccelsTstamp : Outport
  wires:
  In1/1 -> Bus Selector1/1
  Bus Selector1/1 -> Scope2/1, Mux1/1, centripetalTangential/3(w)  "<w>"
  Bus Selector1/5 -> Scope4/1, Mux1/3  "<t>"
  Bus Selector1/3 -> Scope1/1, centripetalTangential/2(ain)  "<a>"
  Logical Operator/1 -> Stop Simulation/1, avoid sending garbage on the last row/2  "all zeros signals end of file"
  Mux1/1 -> Unit Delay/1, avoid sending garbage on the last row/3
  avoid sending garbage on the last row/1 -> gyrosAccelsTstamp/1
  Unit Delay/1 -> avoid sending garbage on the last row/1
  Bus Selector1/2 -> Logical Operator/1, Reshape/1  "<Cbn>"
  Reshape/1 -> centripetalTangential/1(Cbn), Permute Dimensions1/1
  Product/1 -> Mux1/2
  f = a-g/1 -> Product/2
  Constant/1 -> centripetalTangential/5(r)
  Bus Selector1/4 -> Scope3/1, centripetalTangential/4(wdot)  "<wDot>"
  centripetalTangential/1(aout) -> f = a-g/1
  Permute Dimensions1/1 -> Product/1  "Cnb"

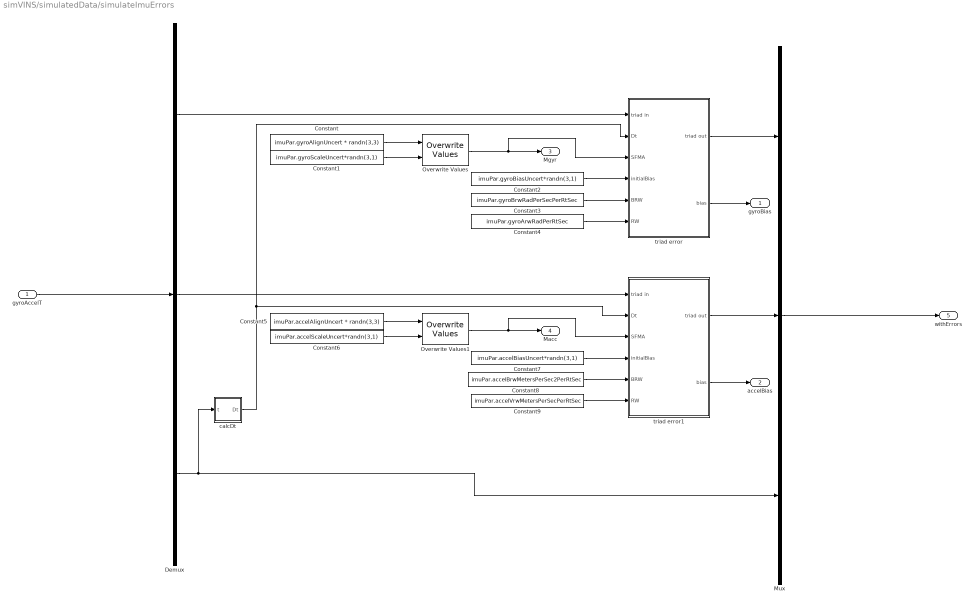
== system simVINS/simulatedData/simulateImuErrors ==
  gyroAccelT : Inport
  Constant : Constant  Value=imuPar.gyroAlignUncert * randn(3,3)
  Constant1 : Constant  Value=imuPar.gyroScaleUncert*randn(3,1)
  Constant2 : Constant  Value=imuPar.gyroBiasUncert*randn(3,1)  VectorParams1D=off
  Constant3 : Constant  Value=imuPar.gyroBrwRadPerSecPerRtSec
  Constant4 : Constant  Value=imuPar.gyroArwRadPerRtSec
  Constant5 : Constant  Value=imuPar.accelAlignUncert * randn(3,3)
  Constant6 : Constant  Value=imuPar.accelScaleUncert*randn(3,1)
  Constant7 : Constant  Value=imuPar.accelBiasUncert*randn(3,1)  VectorParams1D=off
  Constant8 : Constant  Value=imuPar.accelBrwMetersPerSec2PerRtSec
  Constant9 : Constant  Value=imuPar.accelVrwMetersPerSecPerRtSec
  Demux : Demux  Outputs=[3 3 1]
  Mux : Mux  Inputs=3
  Overwrite Values : dspmtrx3/Overwrite Values  OverWriteDiag=Diagonal  valFrom2ndIP=Second input port  ConstValue=0  RowSpan=Range of rows  RowStartMode=First  RowStartIndex=1  RowEndMode=Last  RowEndIndex=1  ColSpan=Range of columns  ColStartMode=First  ColStartIndex=1  ColEndMode=Last  ColEndIndex=1  DiagSpan=All elements  DiagStartMode=Index  DiagStartIndex=2  DiagEndMode=Index  DiagEndIndex=4
      settings: SourceProductName=DSP System Toolbox  SourceProductBaseCode=DS
  Overwrite Values1 : dspmtrx3/Overwrite Values  OverWriteDiag=Diagonal  valFrom2ndIP=Second input port  ConstValue=0  RowSpan=Range of rows  RowStartMode=First  RowStartIndex=1  RowEndMode=Last  RowEndIndex=1  ColSpan=Range of columns  ColStartMode=First  ColStartIndex=1  ColEndMode=Last  ColEndIndex=1  DiagSpan=All elements  DiagStartMode=Index  DiagStartIndex=2  DiagEndMode=Index  DiagEndIndex=4
      settings: SourceProductName=DSP System Toolbox  SourceProductBaseCode=DS
  calcDt : Subsystem
  triad error : Subsystem  TreatAsAtomicUnit=on
  triad error1 : Subsystem  TreatAsAtomicUnit=on
  gyroBias : Outport
  accelBias : Outport  Port=2
  Mgyr : Outport  Port=3
  Macc : Outport  Port=4
  withErrors : Outport  Port=5
  wires:
  gyroAccelT/1 -> Demux/1
  Demux/1 -> triad error/1(triad in)
  triad error/1(triad out) -> Mux/1
  Mux/1 -> withErrors/1
  Constant/1 -> Overwrite Values/1
  Constant1/1 -> Overwrite Values/2
  Overwrite Values/1 -> Mgyr/1, triad error/3(SFMA)
  Constant2/1 -> triad error/4(initialBias)
  triad error/2(bias) -> gyroBias/1
  Constant3/1 -> triad error/5(BRW)
  Constant4/1 -> triad error/6(RW)
  Constant7/1 -> triad error1/4(initialBias)
  Constant9/1 -> triad error1/6(RW)
  Constant8/1 -> triad error1/5(BRW)
  Constant6/1 -> Overwrite Values1/2
  Overwrite Values1/1 -> Macc/1, triad error1/3(SFMA)
  Constant5/1 -> Overwrite Values1/1
  Demux/2 -> triad error1/1(triad in)
  triad error1/1(triad out) -> Mux/2
  triad error1/2(bias) -> accelBias/1
  calcDt/1(Dt) -> triad error1/2(Dt), triad error/2(Dt)
  Demux/3 -> calcDt/1(t), Mux/3

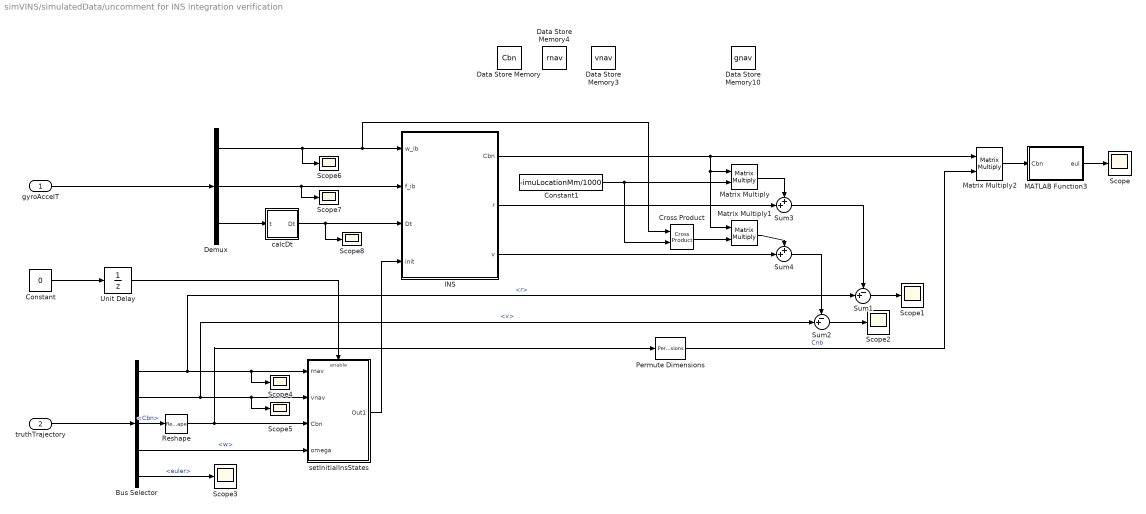
== system simVINS/simulatedData/uncomment for INS integration verification ==
  gyroAccelT : Inport
  truthTrajectory : Inport  Port=2
  Bus Selector : BusSelector  OutputSignals=r,v,Cbn,w,euler
  Constant : Constant  Value=0
  Constant1 : Constant  Value=-imuLocationMm/1000
  Cross Product : vrlib/Utilities/Cross Product
      settings: SourceProductBaseCode=VR
  Data Store Memory : DataStoreMemory  DataStoreName=Cbn  ReadBeforeWriteMsg=warning  WriteAfterWriteMsg=warning  WriteAfterReadMsg=warning  InitialValue=eye(3)  VectorParams1D=off  ShowAdditionalParam=off
  Data Store Memory10 : DataStoreMemory  DataStoreName=gnav  ReadBeforeWriteMsg=warning  WriteAfterWriteMsg=warning  WriteAfterReadMsg=warning  InitialValue=[0;0; 9.80665]  VectorParams1D=off  ShowAdditionalParam=off  OutDataTypeStr=double
  Data Store Memory3 : DataStoreMemory  DataStoreName=vnav  ReadBeforeWriteMsg=warning  WriteAfterWriteMsg=warning  WriteAfterReadMsg=warning  InitialValue=[0;0;0]  VectorParams1D=off  ShowAdditionalParam=off
  Data Store Memory4 : DataStoreMemory  DataStoreName=rnav  ReadBeforeWriteMsg=warning  WriteAfterWriteMsg=warning  WriteAfterReadMsg=warning  InitialValue=[0;0;0]  VectorParams1D=off  ShowAdditionalParam=off
  Demux : Demux  Outputs=[3 3 1]
  INS : Subsystem  Priority=2  TreatAsAtomicUnit=on
      settings: RTWSystemCode=Nonreusable function  RTWFcnNameOpts=Use subsystem name
  MATLAB Function3 : MATLAB Function  TreatAsAtomicUnit=on
  Matrix Multiply : Product  Multiplication=Matrix(*)
  Matrix Multiply1 : Product  Multiplication=Matrix(*)
  Matrix Multiply2 : Product  Multiplication=Matrix(*)
  Permute Dimensions : PermuteDimensions
  Reshape : Reshape  OutputDimensionality=Customize  OutputDimensions=[3,3]
  Scope{,1..8} (9 alike) : Scope
  Sum1 : Sum  Inputs=-+|
  Sum2 : Sum  Inputs=-+|
  Sum3 : Sum  Inputs=++|
  Sum4 : Sum  Inputs=++|
  Unit Delay : UnitDelay  InitialCondition=1  SampleTime=-1
  calcDt : Subsystem
  setInitialInsStates : Subsystem  Priority=1  TreatAsAtomicUnit=on
  wires:
  Demux/3 -> calcDt/1(t)
  gyroAccelT/1 -> Demux/1
  Demux/1 -> Scope6/1, Cross Product/1, INS/1(w_ib)
  Demux/2 -> Scope7/1, INS/2(f_ib)
  calcDt/1(Dt) -> Scope8/1, INS/3(Dt)
  truthTrajectory/1 -> Bus Selector/1
  Bus Selector/1 -> Sum1/2, Scope4/1, setInitialInsStates/1(rnav)  "<r>"
  Bus Selector/2 -> Scope5/1, setInitialInsStates/2(vnav), Sum2/2  "<v>"
  Constant/1 -> Unit Delay/1
  Unit Delay/1 -> setInitialInsStates/Enable
  INS/1(Cbn) -> Matrix Multiply1/1, Matrix Multiply/1, Matrix Multiply2/1
  MATLAB Function3/1(eul) -> Scope/1
  Sum1/1 -> Scope1/1
  Sum3/1 -> Sum1/1
  Sum2/1 -> Scope2/1
  Sum4/1 -> Sum2/1
  Bus Selector/3 -> Reshape/1  "<Cbn>"
  Reshape/1 -> setInitialInsStates/3(Cbn), Permute Dimensions/1
  setInitialInsStates/1(Out1) -> INS/4(init)
  Bus Selector/4 -> setInitialInsStates/4(omega)  "<w>"
  INS/2(r) -> Sum3/2
  Constant1/1 -> Cross Product/2, Matrix Multiply/2
  Matrix Multiply/1 -> Sum3/1
  INS/3(v) -> Sum4/2
  Matrix Multiply1/1 -> Sum4/1
  Cross Product/1 -> Matrix Multiply1/2
  Matrix Multiply2/1 -> MATLAB Function3/1(Cbn)
  Bus Selector/5 -> Scope3/1  "<euler>"
  Permute Dimensions/1 -> Matrix Multiply2/2  "Cnb"

== system simVINS/readFromFile/fetchFeatures/getImgNum ==
  t_us : Inport
  Constant : Constant  Value=imageTstamps
  Gain : Gain  Gain=1000
  Manual Switch : ManualSwitch
  Maximum : dspstat3/Maximum  operation=maximum  fcn=Value and Index  indexBase=One  operateOver=Each column  Dimension=1  InputProcessing=Columns as channels (frame based)  reset=None  roiEnable=off  roiType=Rectangles  roiPortion=Entire ROI  roiOutput=Individual statistics for each ROI  roiFlag=off  roundingMode=Floor  overflowMode=off  accumDataTypeStr=Inherit: Same as product output  accumLastDataTypeStr=Inherit: Same as product output
  Relational Operator : RelationalOperator  Operator===  OutDataTypeStr=boolean  RndMeth=Simplest
  Scope : Scope
  Scope1 : Scope
  imgNum : Outport
  imgFound : Outport  Port=2
  wires:
  Maximum/1 -> imgFound/1
  Gain/1 -> Manual Switch/2  "use picoseconds"
  t_us/1 -> Manual Switch/1, Gain/1  "tstamp_vidcap_us"
  Maximum/2 -> imgNum/1, Scope/1
  Relational Operator/1 -> Maximum/1
  Constant/1 -> Relational Operator/2
  Manual Switch/1 -> Relational Operator/1, Scope1/1

== system simVINS/readFromFile/fetchImages/getImgNum ==
  t_us : Inport
  Constant : Constant  Value=imageTstamps
  Gain : Gain  Gain=1000
  Manual Switch : ManualSwitch
  Maximum : dspstat3/Maximum  operation=maximum  fcn=Value and Index  indexBase=One  operateOver=Each column  Dimension=1  InputProcessing=Columns as channels (frame based)  reset=None  roiEnable=off  roiType=Rectangles  roiPortion=Entire ROI  roiOutput=Individual statistics for each ROI  roiFlag=off  roundingMode=Floor  overflowMode=off  accumDataTypeStr=Inherit: Same as product output  accumLastDataTypeStr=Inherit: Same as product output
  Relational Operator : RelationalOperator  Operator===  OutDataTypeStr=boolean  RndMeth=Simplest
  Scope : Scope
  Scope1 : Scope
  imgNum : Outport
  imgFound : Outport  Port=2
  wires:
  Manual Switch/1 -> Scope1/1, Relational Operator/1
  Constant/1 -> Relational Operator/2
  Relational Operator/1 -> Maximum/1
  Maximum/2 -> Scope/1, imgNum/1
  t_us/1 -> Gain/1, Manual Switch/1  "tstamp_imgPair_us"
  Gain/1 -> Manual Switch/2  "use picoseconds"
  Maximum/1 -> imgFound/1

== system simVINS/simVisionSystem/uncomment and set zero noise and noOverlap for verification/initialize pose ==
  r_b_n : Inport
  C_b_n : Inport  Port=2
  Enable : EnablePort
  Constant : Constant  Value=[0 0 0 1]  VectorParams1D=off
  Data Store Write : DataStoreWrite  DataStoreName=H
  Matrix Concatenate : Concatenate  Mode=Multidimensional array  ConcatenateDimension=2
  Matrix Concatenate1 : Concatenate  Mode=Multidimensional array
  wires:
  Matrix Concatenate1/1 -> Data Store Write/1
  Constant/1 -> Matrix Concatenate1/2
  Matrix Concatenate/1 -> Matrix Concatenate1/1
  r_b_n/1 -> Matrix Concatenate/2
  C_b_n/1 -> Matrix Concatenate/1

== system simVINS/simVisionSystem/uncomment and set zero noise and noOverlap for verification/latch truth pose ==
  r_b_n : Inport
  C_b_n : Inport  Port=2
  pipelineDelayFrames : Inport  Port=3
  Enable : EnablePort
  Delay1 : Delay  DelayLengthSource=Input port
      settings: InputPortMap=u0,p1
  Delay2 : Delay  DelayLengthSource=Input port
      settings: InputPortMap=u0,p1
  rbn : Outport
  Cbn : Outport  Port=2
  wires:
  r_b_n/1 -> Delay1/1
  C_b_n/1 -> Delay2/1
  Delay1/1 -> rbn/1
  Delay2/1 -> Cbn/1
  pipelineDelayFrames/1 -> Delay2/2, Delay1/2

== system simVINS/simVisionSystem/uncomment and set zero noise and noOverlap for verification/plot errors ==
  r_true : Inport
  C_true : Inport  Port=2
  Enable : EnablePort
  Data Store Read : DataStoreRead  DataStoreName=H
  Scope{,1..4} (5 alike) : Scope
  Sum : Sum  Inputs=|+-
  Sum1 : Sum  Inputs=|+-
  extract Cbn : dspmtrx3/Submatrix  RowSpan=Range of rows  RowStartMode=First  RowStartIndex=1  RowEndMode=Index  RowEndIndex=3  ColSpan=Range of columns  ColStartMode=First  ColStartIndex=1  ColEndMode=Index  ColEndIndex=3
  extract r_b_n : dspmtrx3/Submatrix  RowSpan=Range of rows  RowStartMode=First  RowStartIndex=1  RowEndMode=Index  RowEndIndex=3  ColSpan=One column  ColStartMode=Last  ColStartIndex=1  ColEndMode=Index  ColEndIndex=3
  wires:
  Data Store Read/1 -> extract r_b_n/1, extract Cbn/1
  extract r_b_n/1 -> Scope2/1, Sum/1
  r_true/1 -> Scope4/1, Sum/2
  Sum/1 -> Scope/1
  extract Cbn/1 -> Scope3/1, Sum1/1
  C_true/1 -> Sum1/2
  Sum1/1 -> Scope1/1

== system simVINS/simVisionSystem/uncomment and set zero noise and noOverlap for verification/update pose ==
  r_2_1 : Inport
  C_2_1 : Inport  Port=2
  Enable : EnablePort
  Constant : Constant  Value=[0 0 0 1]  VectorParams1D=off
  Data Store Read : DataStoreRead  DataStoreName=H
  Data Store Write : DataStoreWrite  DataStoreName=H
  Matrix Concatenate : Concatenate  Mode=Multidimensional array  ConcatenateDimension=2
  Matrix Concatenate1 : Concatenate  Mode=Multidimensional array
  Matrix Multiply : Product  Multiplication=Matrix(*)
  wires:
  C_2_1/1 -> Matrix Concatenate/1
  r_2_1/1 -> Matrix Concatenate/2
  Matrix Concatenate/1 -> Matrix Concatenate1/1
  Constant/1 -> Matrix Concatenate1/2
  Data Store Read/1 -> Matrix Multiply/1
  Matrix Concatenate1/1 -> Matrix Multiply/2
  Matrix Multiply/1 -> Data Store Write/1
